simulink library "csc_vac_vernier_acs_ctrl_lib"  (R2015b)
settings: Solver=ode45  StartTime=0.0  StopTime=10.0  RelTol=1e-3
values from neighbouring files (symbols this model uses):
  vac_alpha_gain = 0.2    [csc_vac_vernier_acs_ctrl_init.m]
  vac_rotx_deadband = 1*pi/180    (= 0.0174532925199)    [csc_vac_vernier_acs_ctrl_init.m]
  vac_rotx_deadband_minus = 1*pi/180    (= 0.0174532925199)    [csc_vac_vernier_acs_ctrl_init.m]
  vac_roty_deadband = 1*pi/180    (= 0.0174532925199)    [csc_vac_vernier_acs_ctrl_init.m]
  vac_roty_deadband_minus = 1*pi/180    (= 0.0174532925199)    [csc_vac_vernier_acs_ctrl_init.m]
  vac_rotz_deadband = 1*pi/180    (= 0.0174532925199)    [csc_vac_vernier_acs_ctrl_init.m]
  vac_rotz_deadband_minus = 1*pi/180    (= 0.0174532925199)    [csc_vac_vernier_acs_ctrl_init.m]
  vac_thruster_alloc_vernier_x_minus = [16,24]    [csc_vac_vernier_acs_ctrl_init.m]
  vac_thruster_alloc_vernier_x_plus = [18,22]    [csc_vac_vernier_acs_ctrl_init.m]
  vac_thruster_alloc_vernier_y_minus = [15,19]    [csc_vac_vernier_acs_ctrl_init.m]
  vac_thruster_alloc_vernier_y_plus = [13,21]    [csc_vac_vernier_acs_ctrl_init.m]
  vac_thruster_alloc_vernier_z_minus = [14,20]    [csc_vac_vernier_acs_ctrl_init.m]
  vac_thruster_alloc_vernier_z_plus = [17,23]    [csc_vac_vernier_acs_ctrl_init.m]
undefined symbols (not defined in the file or in its folder): csc_cnt_dt, emp_inertia_wet_dry, emp_mass_wet_dry, vac_vernier_thruster_trq_x, vac_vernier_thruster_trq_y, vac_vernier_thruster_trq_z
libraries: csu_ppd_phase_plane_distance_lib x3, util_info_lib x1, csu_ptc_vernier_phaseplane_thruster_alloc_lib x1
settings Model: Creator=Nilesh  LastModifiedBy=jimkaidy
settings DataIOCC: SaveFormat=Array
settings DebuggingCC: UnderspecifiedInitializationDetection=Classic  MergeDetectMultiDrivingBlocksExec=none  SolverPrmCheckMsg=warning  StateNameClashWarn=warning
settings HardwareCC: ProdBitPerPointer=32  ProdLargestAtomicFloat=None  ProdIntDivRoundTo=Undefined  ProdEndianess=Unspecified  ProdWordSize=32  ProdHWDeviceType=32-bit Generic
settings GRTTargetCC: GeneratePreprocessorConditionals=Disable all
settings ConfigComp: CovModelRefEnable=Off  CovSFcnEnable=off

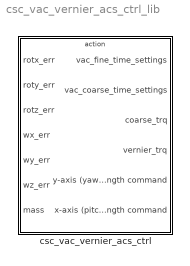
== system csc_vac_vernier_acs_ctrl_lib ==
  csc_vac_vernier_acs_ctrl : Subsystem

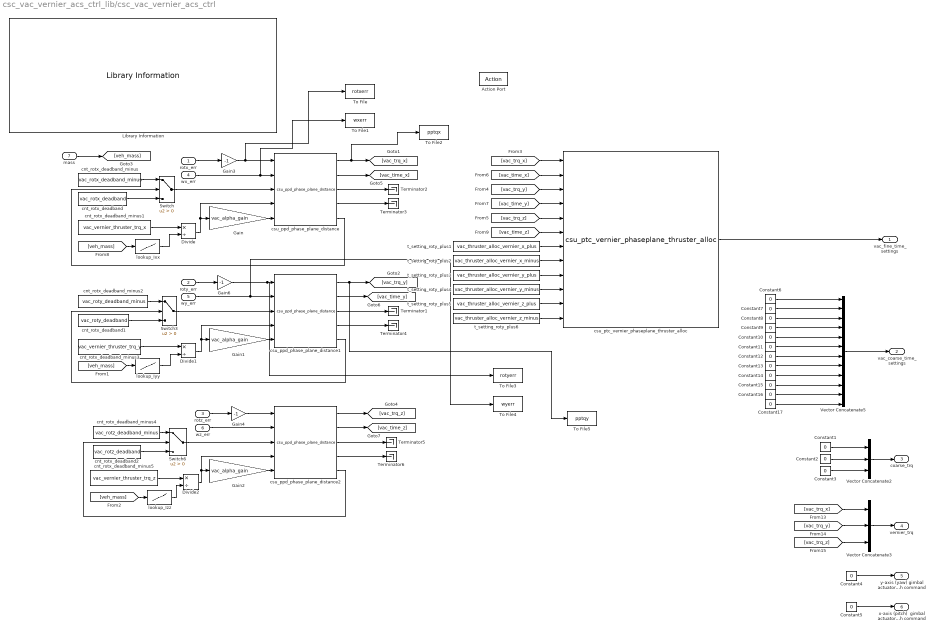
== system csc_vac_vernier_acs_ctrl_lib/csc_vac_vernier_acs_ctrl ==
  rotx_err : Inport
  roty_err : Inport  Port=2
  rotz_err : Inport  Port=3
  wx_err : Inport  Port=4
  wy_err : Inport  Port=5
  wz_err : Inport  Port=6
  mass : Inport  Port=7
  Action Port : ActionPort
  Constant1 : Constant  Value=0  OutDataTypeStr=int8  SampleTime=csc_cnt_dt
  Constant{6..17} (12 alike) : Constant  Value=0  OutDataTypeStr=uint8  SampleTime=csc_cnt_dt
  Constant2 : Constant  Value=0  OutDataTypeStr=int8  SampleTime=csc_cnt_dt
  Constant3 : Constant  Value=0  OutDataTypeStr=int8  SampleTime=csc_cnt_dt
  Constant4 : Constant  Value=0  OutDataTypeStr=double
  Constant5 : Constant  Value=0  OutDataTypeStr=double
  Divide : Product  Inputs=*/
  Divide1 : Product  Inputs=*/
  Divide2 : Product  Inputs=*/
  Gain : Gain  Gain=vac_alpha_gain
  Gain1 : Gain  Gain=vac_alpha_gain
  Gain2 : Gain  Gain=vac_alpha_gain
  Gain3 : Gain  Gain=-1
  Gain4 : Gain  Gain=-1
  Gain6 : Gain  Gain=-1
  Library Information : util_info_lib/Library Information  owner='NONE'
  Switch : Switch  Criteria=u2 > Threshold
  Switch3 : Switch  Criteria=u2 > Threshold
  Switch6 : Switch  Criteria=u2 > Threshold
  Terminator{1..6} (6 alike) : Terminator
  To File : ToFile  Filename=rotxerr  MatrixName=rotxerr  SaveFormat=Timeseries
  To File1 : ToFile  Filename=wxerr  MatrixName=wxerr  SaveFormat=Timeseries
  To File2 : ToFile  Filename=pptqx  MatrixName=pptqx  SaveFormat=Timeseries
  To File3 : ToFile  Filename=rotyerr  MatrixName=rotyerr  SaveFormat=Timeseries
  To File4 : ToFile  Filename=wyerr  MatrixName=wyerr  SaveFormat=Timeseries
  To File5 : ToFile  Filename=pptqy  MatrixName=pptqy  SaveFormat=Timeseries
  Vector Concatenate2 : Concatenate  NumInputs=3
  Vector Concatenate3 : Concatenate  NumInputs=3
  Vector Concatenate5 : Concatenate  NumInputs=12
  cnt_rotx_deadband : Constant  Value=vac_rotx_deadband
  cnt_rotx_deadband1 : Constant  Value=vac_roty_deadband
  cnt_rotx_deadband2 : Constant  Value=vac_rotz_deadband
  cnt_rotx_deadband_minus : Constant  Value=vac_rotx_deadband_minus
  cnt_rotx_deadband_minus1 : Constant  Value=vac_vernier_thruster_trq_x
  cnt_rotx_deadband_minus2 : Constant  Value=vac_roty_deadband_minus
  cnt_rotx_deadband_minus3 : Constant  Value=vac_vernier_thruster_trq_y
  cnt_rotx_deadband_minus4 : Constant  Value=vac_rotz_deadband_minus
  cnt_rotx_deadband_minus5 : Constant  Value=vac_vernier_thruster_trq_z
  csu_ppd_phase_plane_distance : csu_ppd_phase_plane_distance_lib/csu_ppd_phase_plane_distance
  csu_ppd_phase_plane_distance1 : csu_ppd_phase_plane_distance_lib/csu_ppd_phase_plane_distance
  csu_ppd_phase_plane_distance2 : csu_ppd_phase_plane_distance_lib/csu_ppd_phase_plane_distance
  csu_ptc_vernier_phaseplane_thruster_alloc : csu_ptc_vernier_phaseplane_thruster_alloc_lib/csu_ptc_vernier_phaseplane_thruster_alloc
  lookup_Ixx : Lookup  InputValues=emp_mass_wet_dry  Table=emp_inertia_wet_dry(1,:)
  lookup_Iyy : Lookup  InputValues=emp_mass_wet_dry  Table=emp_inertia_wet_dry(2,:)
  lookup_Izz : Lookup  InputValues=emp_mass_wet_dry  Table=emp_inertia_wet_dry(3,:)
  t_setting_roty_plus1 : Constant  Value=vac_thruster_alloc_vernier_x_plus
  t_setting_roty_plus2 : Constant  Value=vac_thruster_alloc_vernier_x_minus
  t_setting_roty_plus3 : Constant  Value=vac_thruster_alloc_vernier_y_plus
  t_setting_roty_plus4 : Constant  Value=vac_thruster_alloc_vernier_y_minus
  t_setting_roty_plus5 : Constant  Value=vac_thruster_alloc_vernier_z_plus
  t_setting_roty_plus6 : Constant  Value=vac_thruster_alloc_vernier_z_minus
  vac_fine_time_settings : Outport
  vac_coarse_time_settings : Outport  Port=2
  coarse_trq : Outport  Port=3
  vernier_trq : Outport  Port=4
  y-axis (yaw) gimbal actuator langth command : Outport  Port=5
  x-axis (pitch)  gimbal actuator langth command : Outport  Port=6
  wires:
  Vector Concatenate5/1 -> vac_coarse_time_settings/1
  Constant12/1 -> Vector Concatenate5/7
  Constant13/1 -> Vector Concatenate5/8
  Constant11/1 -> Vector Concatenate5/6
  Constant10/1 -> Vector Concatenate5/5
  Constant14/1 -> Vector Concatenate5/9
  Constant15/1 -> Vector Concatenate5/10
  Constant9/1 -> Vector Concatenate5/4
  Constant8/1 -> Vector Concatenate5/3
  Constant16/1 -> Vector Concatenate5/11
  Constant7/1 -> Vector Concatenate5/2
  Constant17/1 -> Vector Concatenate5/12
  Constant6/1 -> Vector Concatenate5/1
  [vac_trq_x] -> Vector Concatenate3/1
  [vac_trq_y] -> Vector Concatenate3/2
  Vector Concatenate3/1 -> vernier_trq/1
  [vac_trq_z] -> Vector Concatenate3/3
  Constant1/1 -> Vector Concatenate2/1
  Constant2/1 -> Vector Concatenate2/2
  Vector Concatenate2/1 -> coarse_trq/1
  Constant3/1 -> Vector Concatenate2/3
  Divide1/1 -> csu_ppd_phase_plane_distance1/4, Gain1/1
  Gain/1 -> csu_ppd_phase_plane_distance/5
  Divide/1 -> Gain/1, csu_ppd_phase_plane_distance/4
  Switch/1 -> csu_ppd_phase_plane_distance/3
  cnt_rotx_deadband/1 -> Switch/3
  cnt_rotx_deadband_minus/1 -> Switch/1
  csu_ppd_phase_plane_distance/5 -> Switch/2
  wx_err/1 -> To File1/1, csu_ppd_phase_plane_distance/2
  rotx_err/1 -> Gain3/1
  Switch3/1 -> csu_ppd_phase_plane_distance1/3
  wy_err/1 -> To File4/1, csu_ppd_phase_plane_distance1/2
  roty_err/1 -> Gain6/1
  rotz_err/1 -> Gain4/1
  wz_err/1 -> csu_ppd_phase_plane_distance2/2
  mass/1 -> [veh_mass]
  [veh_mass] -> lookup_Ixx/1
  lookup_Ixx/1 -> Divide/2
  cnt_rotx_deadband_minus1/1 -> Divide/1
  cnt_rotx_deadband1/1 -> Switch3/3
  cnt_rotx_deadband_minus2/1 -> Switch3/1
  csu_ppd_phase_plane_distance1/5 -> Switch3/2
  [veh_mass] -> lookup_Iyy/1
  lookup_Iyy/1 -> Divide1/2
  cnt_rotx_deadband_minus3/1 -> Divide1/1
  Gain1/1 -> csu_ppd_phase_plane_distance1/5
  Switch6/1 -> csu_ppd_phase_plane_distance2/3
  cnt_rotx_deadband2/1 -> Switch6/3
  cnt_rotx_deadband_minus4/1 -> Switch6/1
  csu_ppd_phase_plane_distance2/5 -> Switch6/2
  [veh_mass] -> lookup_Izz/1
  lookup_Izz/1 -> Divide2/2
  cnt_rotx_deadband_minus5/1 -> Divide2/1
  Divide2/1 -> Gain2/1, csu_ppd_phase_plane_distance2/4
  Gain2/1 -> csu_ppd_phase_plane_distance2/5
  csu_ppd_phase_plane_distance/1 -> To File2/1, [vac_trq_x]
  csu_ppd_phase_plane_distance2/1 -> [vac_trq_z]
  Gain6/1 -> To File3/1, csu_ppd_phase_plane_distance1/1
  Gain3/1 -> To File/1, csu_ppd_phase_plane_distance/1
  Gain4/1 -> csu_ppd_phase_plane_distance2/1
  csu_ppd_phase_plane_distance/2 -> [vac_time_x]
  csu_ppd_phase_plane_distance1/2 -> [vac_time_y]
  csu_ppd_phase_plane_distance2/2 -> [vac_time_z]
  [vac_trq_x] -> csu_ptc_vernier_phaseplane_thruster_alloc/1
  [vac_trq_y] -> csu_ptc_vernier_phaseplane_thruster_alloc/3
  [vac_trq_z] -> csu_ptc_vernier_phaseplane_thruster_alloc/5
  t_setting_roty_plus1/1 -> csu_ptc_vernier_phaseplane_thruster_alloc/7
  t_setting_roty_plus2/1 -> csu_ptc_vernier_phaseplane_thruster_alloc/8
  t_setting_roty_plus3/1 -> csu_ptc_vernier_phaseplane_thruster_alloc/9
  t_setting_roty_plus4/1 -> csu_ptc_vernier_phaseplane_thruster_alloc/10
  t_setting_roty_plus5/1 -> csu_ptc_vernier_phaseplane_thruster_alloc/11
  t_setting_roty_plus6/1 -> csu_ptc_vernier_phaseplane_thruster_alloc/12
  [vac_time_x] -> csu_ptc_vernier_phaseplane_thruster_alloc/2
  [vac_time_z] -> csu_ptc_vernier_phaseplane_thruster_alloc/6
  [vac_time_y] -> csu_ptc_vernier_phaseplane_thruster_alloc/4
  csu_ptc_vernier_phaseplane_thruster_alloc/1 -> vac_fine_time_settings/1
  csu_ppd_phase_plane_distance/4 -> Terminator3/1
  csu_ppd_phase_plane_distance/3 -> Terminator2/1
  csu_ppd_phase_plane_distance2/4 -> Terminator6/1
  csu_ppd_phase_plane_distance2/3 -> Terminator5/1
  csu_ppd_phase_plane_distance1/4 -> Terminator4/1
  csu_ppd_phase_plane_distance1/3 -> Terminator1/1
  Constant5/1 -> x-axis (pitch)  gimbal actuator langth command/1
  Constant4/1 -> y-axis (yaw) gimbal actuator langth command/1
  csu_ppd_phase_plane_distance1/1 -> To File5/1, [vac_trq_y]
